simulink model "viertanksystempidstoer"  (Simulink 3.00)
settings: Solver=ode45  StartTime=0.0  StopTime=1800  FixedStep=0.01  RelTol=1e-6  AbsTol=1e-6
undefined symbols (not defined in the file or in its folder): A, A12, A23, A34, A4, g, TN, TV
libraries: simulink3 x1
settings Model: SaveTime=off  SaveOutput=off

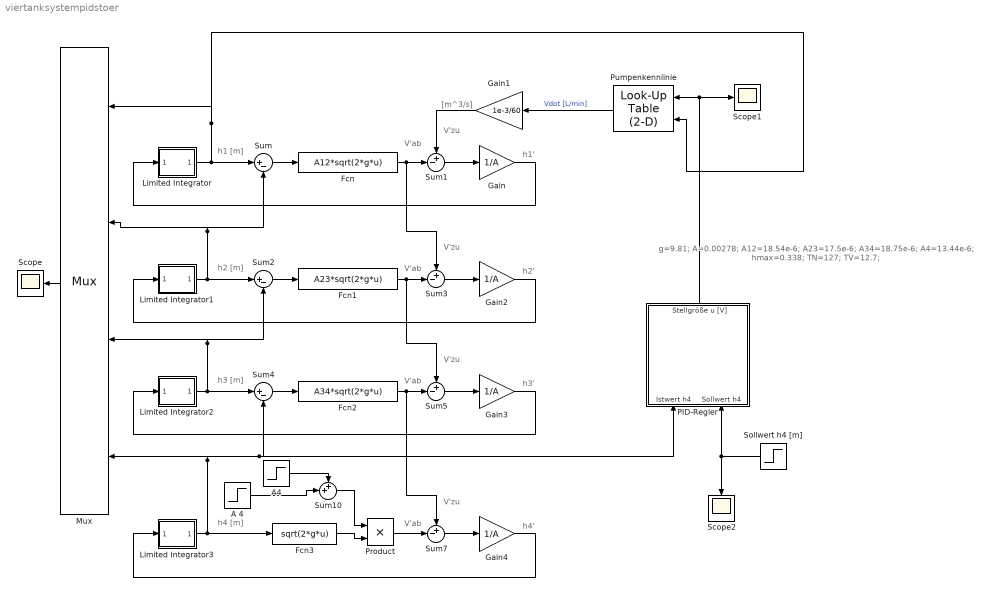
== system viertanksystempidstoer ==
  note: h1 [m]
  note: h1'
  note: [m^3/s]
  note: g=9.81;
      | A=0.00278;
      | A12=18.54e-6;
      | A23=17.5e-6;
      | A34=18.75e-6;
      | A4=13.44e-6;
      | hmax=0.338;
      | TN=127;
      | TV=12.7;
  note: h2 [m]
  note: h2'
  note: V'zu
  note: V'ab
  note: V'zu
  note: V'ab
  note: h3 [m]
  note: h3'
  note: V'zu
  note: V'ab
  note: h4 [m]
  note: h4'
  note: V'zu
  note: V'ab
  A 4 : Step  Time=1230  Before=0  After=A4*0.1749  SampleTime=0
  A4 : Step  Time=600  Before=A4  After=A4*0.8251  SampleTime=0
  Fcn : Fcn  Expr=A12*sqrt(2*g*u)
  Fcn1 : Fcn  Expr=A23*sqrt(2*g*u)
  Fcn2 : Fcn  Expr=A34*sqrt(2*g*u)
  Fcn3 : Fcn  Expr=sqrt(2*g*u)
  Gain{,2..4} (4 alike) : Gain  Gain=1/A  SaturateOnIntegerOverflow=on
  Gain1 : Gain  Orientation=left  Gain=1e-3/60  SaturateOnIntegerOverflow=on
  Limited Integrator : Subsystem  mask(Limited Integrator.){@1=0, @2=hmax, @3=0}
      mask prompts: @1 "Lower bound:"; @2 "Upper bound:"; @3 "Initial condition:"
      mask help: Limited Integrator
      mask init:
      | lower_limit=@1;upper_limit=@2;X0=@3;
      mask Help: Implements a limited integrator with \nan expression of the form:\n\nif(x<=lb and u<0) or (x>=ub and u>0)\n   xdot=0\nelse\n   xdot=u
      mask Display: plot(-1,-0.2,3.5,1.2,[0.05,1,2,2.9],[0,0,1,1]);disp(' 1/s    ')
  Limited Integrator1 : Subsystem  mask(Limited Integrator.){@1=0, @2=hmax, @3=0}
      mask prompts: @1 "Lower bound:"; @2 "Upper bound:"; @3 "Initial condition:"
      mask help: Limited Integrator
      mask init:
      | lower_limit=@1;upper_limit=@2;X0=@3;
      mask Help: Implements a limited integrator with \nan expression of the form:\n\nif(x<=lb and u<0) or (x>=ub and u>0)\n   xdot=0\nelse\n   xdot=u
      mask Display: plot(-1,-0.2,3.5,1.2,[0.05,1,2,2.9],[0,0,1,1]);disp(' 1/s    ')
  Limited Integrator2 : Subsystem  mask(Limited Integrator.){@1=0, @2=hmax, @3=0}
      mask prompts: @1 "Lower bound:"; @2 "Upper bound:"; @3 "Initial condition:"
      mask help: Limited Integrator
      mask init:
      | lower_limit=@1;upper_limit=@2;X0=@3;
      mask Help: Implements a limited integrator with \nan expression of the form:\n\nif(x<=lb and u<0) or (x>=ub and u>0)\n   xdot=0\nelse\n   xdot=u
      mask Display: plot(-1,-0.2,3.5,1.2,[0.05,1,2,2.9],[0,0,1,1]);disp(' 1/s    ')
  Limited Integrator3 : Subsystem  mask(Limited Integrator.){@1=0, @2=hmax, @3=0}
      mask prompts: @1 "Lower bound:"; @2 "Upper bound:"; @3 "Initial condition:"
      mask help: Limited Integrator
      mask init:
      | lower_limit=@1;upper_limit=@2;X0=@3;
      mask Help: Implements a limited integrator with \nan expression of the form:\n\nif(x<=lb and u<0) or (x>=ub and u>0)\n   xdot=0\nelse\n   xdot=u
      mask Display: plot(-1,-0.2,3.5,1.2,[0.05,1,2,2.9],[0,0,1,1]);disp(' 1/s    ')
  Mux : Mux  Orientation=left  Inputs=4
      settings: DisplayOption=none
  PID-Regler : Subsystem  Orientation=up
  Product : Product  Inputs=2  SaturateOnIntegerOverflow=on
  Pumpenkennlinie : simulink3/Functions & Tables/Look-Up Table (2-D)  Orientation=left  x=[ 0 2 3.5 4 6 8 10 12]  y=[ 0 1 2 3 4 5 6 7 8 9 10]*0.338/10  t=[ 0 0 0 0 0 0 0 0 0 0 0 ; 0 0 0 0 0 0 0 0 0 0 0 ; 0.3373 0.2611 0.1115 0.0311 0 0 0 0 0 0 0 ; 0.6051 0.5588 0.5222 0.4851 0.4488 0.3499 0.2844 0.2148 0.1899 0.1431 0.0861; 1.3367 1.3073 1.2845 1.2640 1.2531 1.2297 1.2081 1.1914 1.1831 1.1704 1.1614 ; 1.8718 1.8689 1.8632 1.8579 1.8491 1.8375 1.8271 1.8120 1.8045 1.7843 1.7733 ; 2.4327 2.4253 2.4193 2.4161 2.4095 2.4071 2.4035 2.3993 2.3941 2.3847 2.3799 ; 2.9356 2.9306 2.9291 2.9187 2.9165 2.9125 2.8945 2.8922 2.8855 2.8775 2.8744 ]
  Scope : Scope
      settings: TimeRange=auto  YMin=0.08  YMax=0.18  SaveName=h  DataFormat=Matrix
  Scope1 : Scope
      settings: TimeRange=auto  YMin=7e-034  YMax=2.1e-033  SaveName=up  DataFormat=Matrix
  Scope2 : Scope
      settings: Orientation=down  TimeRange=auto  YMin=-1  YMax=1.1  SaveName=w  DataFormat=Matrix
  Sollwert h4 [m] : Step  Orientation=left  Time=5  Before=0  After=2.5*0.0338  SampleTime=0
  Sum : Sum  Inputs=|+-  SaturateOnIntegerOverflow=on
  Sum{1,3,5,7} (4 alike) : Sum  Inputs=+-|  SaturateOnIntegerOverflow=on
  Sum10 : Sum  Inputs=++|  SaturateOnIntegerOverflow=on
  Sum2 : Sum  Inputs=|+-  SaturateOnIntegerOverflow=on
  Sum4 : Sum  Inputs=|+-  SaturateOnIntegerOverflow=on
  wires:
  Sum/1 -> Fcn/1
  Limited Integrator/1(Outport) -> Sum/1, Mux/1, Pumpenkennlinie/2
  Sum1/1 -> Gain/1
  Gain/1 -> Limited Integrator/1(Inport)
  Gain1/1 -> Sum1/1
  Sum2/1 -> Fcn1/1
  Sum3/1 -> Gain2/1
  Gain2/1 -> Limited Integrator1/1(Inport)
  Limited Integrator1/1(Outport) -> Sum2/1, Sum/2, Mux/2
  Fcn/1 -> Sum1/2, Sum3/1
  Sum4/1 -> Fcn2/1
  Sum5/1 -> Gain3/1
  Gain3/1 -> Limited Integrator2/1(Inport)
  Limited Integrator2/1(Outport) -> Sum4/1, Sum2/2, Mux/3
  Fcn2/1 -> Sum5/2, Sum7/1
  Fcn1/1 -> Sum3/2, Sum5/1
  Pumpenkennlinie/1 -> Gain1/1  "Vdot [L/min]"
  Mux/1 -> Scope/1
  Sum7/1 -> Gain4/1
  Gain4/1 -> Limited Integrator3/1(Inport)
  Limited Integrator3/1(Outport) -> Fcn3/1, Mux/4, Sum4/2, PID-Regler/1(Istwert h4)
  Fcn3/1 -> Product/2
  Product/1 -> Sum7/2
  A4/1 -> Sum10/1
  A 4/1 -> Sum10/2
  Sum10/1 -> Product/1
  PID-Regler/1(Stellgröße u [V]) -> Pumpenkennlinie/1, Scope1/1
  Sollwert h4 [m]/1 -> PID-Regler/2(Sollwert h4), Scope2/1

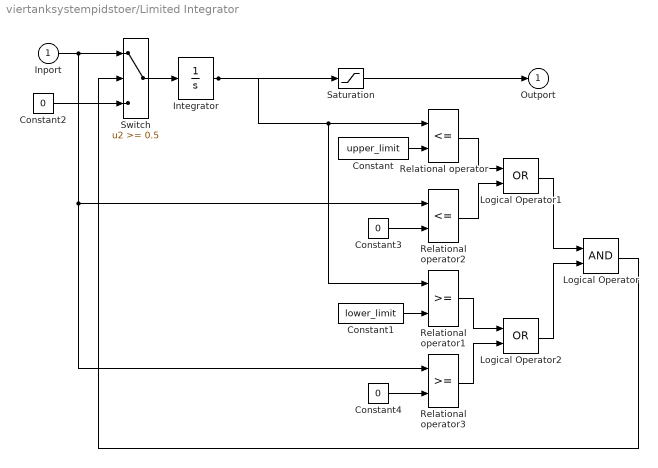
== system viertanksystempidstoer/Limited Integrator ==
  Inport : Inport  Port=1  PortWidth=-1  SampleTime=-1  DataType=auto
      settings: SignalType=auto
  Constant : Constant  Value=upper_limit
  Constant1 : Constant  Value=lower_limit
  Constant2 : Constant  Value=0
  Constant3 : Constant  Value=0
  Constant4 : Constant  Value=0
  Integrator : Integrator  ExternalReset=none  InitialConditionSource=internal  InitialCondition=X0  LimitOutput=off  UpperSaturationLimit=inf  LowerSaturationLimit=-inf  ShowSaturationPort=off  ShowStatePort=off  AbsoluteTolerance=auto
  Logical Operator : Logic  Operator=AND  Inputs=2
  Logical Operator1 : Logic  Operator=OR  Inputs=2
  Logical Operator2 : Logic  Operator=OR  Inputs=2
  Relational operator : RelationalOperator  Operator=<=
  Relational operator1 : RelationalOperator  Operator=>=
  Relational operator2 : RelationalOperator  Operator=<=
  Relational operator3 : RelationalOperator  Operator=>=
  Saturation : Saturate  UpperLimit=upper_limit  LowerLimit=lower_limit
  Switch : Switch  Threshold=0.5
  Outport : Outport  Port=1
  wires:
  Saturation/1 -> Outport/1
  Inport/1 -> Switch/1, Relational operator2/1, Relational operator3/1
  Switch/1 -> Integrator/1
  Constant/1 -> Relational operator/2
  Constant1/1 -> Relational operator1/2
  Logical Operator/1 -> Switch/2
  Constant2/1 -> Switch/3
  Relational operator/1 -> Logical Operator1/1
  Relational operator2/1 -> Logical Operator1/2
  Logical Operator1/1 -> Logical Operator/1
  Relational operator1/1 -> Logical Operator2/1
  Relational operator3/1 -> Logical Operator2/2
  Logical Operator2/1 -> Logical Operator/2
  Constant3/1 -> Relational operator2/2
  Constant4/1 -> Relational operator3/2
  Integrator/1 -> Saturation/1, Relational operator1/1, Relational operator/1

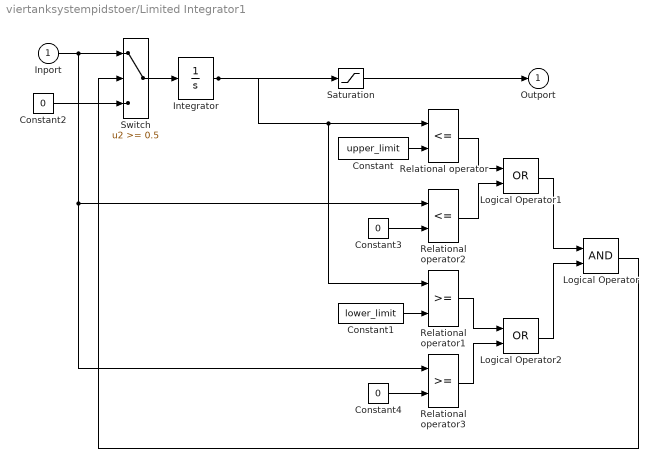
== system viertanksystempidstoer/Limited Integrator1 ==
  Inport : Inport  Port=1  PortWidth=-1  SampleTime=-1  DataType=auto
      settings: SignalType=auto
  Constant : Constant  Value=upper_limit
  Constant1 : Constant  Value=lower_limit
  Constant2 : Constant  Value=0
  Constant3 : Constant  Value=0
  Constant4 : Constant  Value=0
  Integrator : Integrator  ExternalReset=none  InitialConditionSource=internal  InitialCondition=X0  LimitOutput=off  UpperSaturationLimit=inf  LowerSaturationLimit=-inf  ShowSaturationPort=off  ShowStatePort=off  AbsoluteTolerance=auto
  Logical Operator : Logic  Operator=AND  Inputs=2
  Logical Operator1 : Logic  Operator=OR  Inputs=2
  Logical Operator2 : Logic  Operator=OR  Inputs=2
  Relational operator : RelationalOperator  Operator=<=
  Relational operator1 : RelationalOperator  Operator=>=
  Relational operator2 : RelationalOperator  Operator=<=
  Relational operator3 : RelationalOperator  Operator=>=
  Saturation : Saturate  UpperLimit=upper_limit  LowerLimit=lower_limit
  Switch : Switch  Threshold=0.5
  Outport : Outport  Port=1
  wires:
  Integrator/1 -> Relational operator/1, Relational operator1/1, Saturation/1
  Constant4/1 -> Relational operator3/2
  Constant3/1 -> Relational operator2/2
  Logical Operator2/1 -> Logical Operator/2
  Relational operator3/1 -> Logical Operator2/2
  Relational operator1/1 -> Logical Operator2/1
  Logical Operator1/1 -> Logical Operator/1
  Relational operator2/1 -> Logical Operator1/2
  Relational operator/1 -> Logical Operator1/1
  Constant2/1 -> Switch/3
  Logical Operator/1 -> Switch/2
  Constant1/1 -> Relational operator1/2
  Constant/1 -> Relational operator/2
  Switch/1 -> Integrator/1
  Inport/1 -> Relational operator3/1, Relational operator2/1, Switch/1
  Saturation/1 -> Outport/1

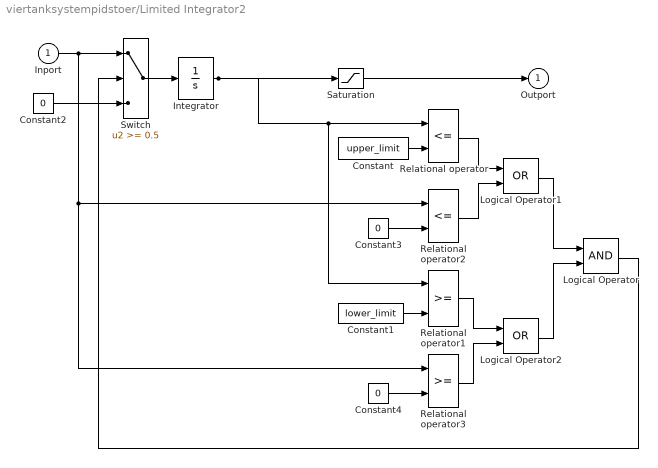
== system viertanksystempidstoer/Limited Integrator2 ==
  Inport : Inport  Port=1  PortWidth=-1  SampleTime=-1  DataType=auto
      settings: SignalType=auto
  Constant : Constant  Value=upper_limit
  Constant1 : Constant  Value=lower_limit
  Constant2 : Constant  Value=0
  Constant3 : Constant  Value=0
  Constant4 : Constant  Value=0
  Integrator : Integrator  ExternalReset=none  InitialConditionSource=internal  InitialCondition=X0  LimitOutput=off  UpperSaturationLimit=inf  LowerSaturationLimit=-inf  ShowSaturationPort=off  ShowStatePort=off  AbsoluteTolerance=auto
  Logical Operator : Logic  Operator=AND  Inputs=2
  Logical Operator1 : Logic  Operator=OR  Inputs=2
  Logical Operator2 : Logic  Operator=OR  Inputs=2
  Relational operator : RelationalOperator  Operator=<=
  Relational operator1 : RelationalOperator  Operator=>=
  Relational operator2 : RelationalOperator  Operator=<=
  Relational operator3 : RelationalOperator  Operator=>=
  Saturation : Saturate  UpperLimit=upper_limit  LowerLimit=lower_limit
  Switch : Switch  Threshold=0.5
  Outport : Outport  Port=1
  wires:
  Saturation/1 -> Outport/1
  Inport/1 -> Switch/1, Relational operator2/1, Relational operator3/1
  Switch/1 -> Integrator/1
  Constant/1 -> Relational operator/2
  Constant1/1 -> Relational operator1/2
  Logical Operator/1 -> Switch/2
  Constant2/1 -> Switch/3
  Relational operator/1 -> Logical Operator1/1
  Relational operator2/1 -> Logical Operator1/2
  Logical Operator1/1 -> Logical Operator/1
  Relational operator1/1 -> Logical Operator2/1
  Relational operator3/1 -> Logical Operator2/2
  Logical Operator2/1 -> Logical Operator/2
  Constant3/1 -> Relational operator2/2
  Constant4/1 -> Relational operator3/2
  Integrator/1 -> Saturation/1, Relational operator1/1, Relational operator/1

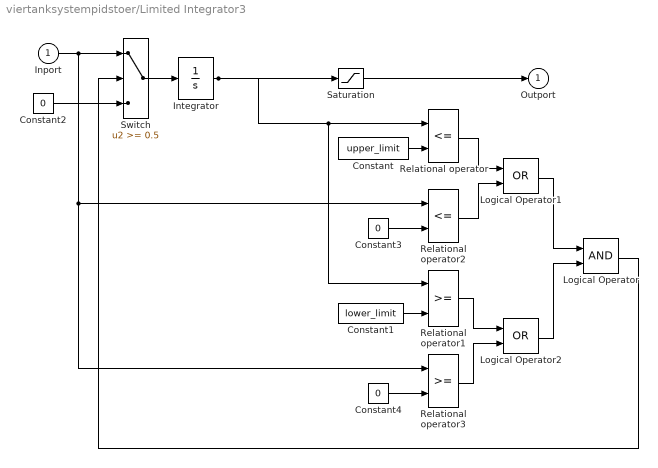
== system viertanksystempidstoer/Limited Integrator3 ==
  Inport : Inport  Port=1  PortWidth=-1  SampleTime=-1  DataType=auto
      settings: SignalType=auto
  Constant : Constant  Value=upper_limit
  Constant1 : Constant  Value=lower_limit
  Constant2 : Constant  Value=0
  Constant3 : Constant  Value=0
  Constant4 : Constant  Value=0
  Integrator : Integrator  ExternalReset=none  InitialConditionSource=internal  InitialCondition=X0  LimitOutput=off  UpperSaturationLimit=inf  LowerSaturationLimit=-inf  ShowSaturationPort=off  ShowStatePort=off  AbsoluteTolerance=auto
  Logical Operator : Logic  Operator=AND  Inputs=2
  Logical Operator1 : Logic  Operator=OR  Inputs=2
  Logical Operator2 : Logic  Operator=OR  Inputs=2
  Relational operator : RelationalOperator  Operator=<=
  Relational operator1 : RelationalOperator  Operator=>=
  Relational operator2 : RelationalOperator  Operator=<=
  Relational operator3 : RelationalOperator  Operator=>=
  Saturation : Saturate  UpperLimit=upper_limit  LowerLimit=lower_limit
  Switch : Switch  Threshold=0.5
  Outport : Outport  Port=1
  wires:
  Integrator/1 -> Relational operator/1, Relational operator1/1, Saturation/1
  Constant4/1 -> Relational operator3/2
  Constant3/1 -> Relational operator2/2
  Logical Operator2/1 -> Logical Operator/2
  Relational operator3/1 -> Logical Operator2/2
  Relational operator1/1 -> Logical Operator2/1
  Logical Operator1/1 -> Logical Operator/1
  Relational operator2/1 -> Logical Operator1/2
  Relational operator/1 -> Logical Operator1/1
  Constant2/1 -> Switch/3
  Logical Operator/1 -> Switch/2
  Constant1/1 -> Relational operator1/2
  Constant/1 -> Relational operator/2
  Switch/1 -> Integrator/1
  Inport/1 -> Relational operator3/1, Relational operator2/1, Switch/1
  Saturation/1 -> Outport/1

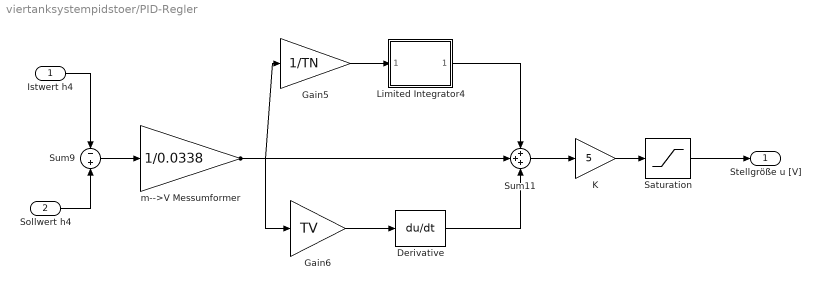
== system viertanksystempidstoer/PID-Regler ==
  Istwert h4 : Inport  Port=1  PortWidth=-1  SampleTime=-1  DataType=auto
      settings: SignalType=auto
  Sollwert h4 : Inport  Port=2  PortWidth=-1  SampleTime=-1  DataType=auto
      settings: SignalType=auto
  Derivative : Derivative
  Gain5 : Gain  Gain=1/TN  SaturateOnIntegerOverflow=on
  Gain6 : Gain  Gain=TV  SaturateOnIntegerOverflow=on
  K : Gain  Gain=5  SaturateOnIntegerOverflow=on
  Limited Integrator4 : Subsystem  mask(Limited Integrator.){@1=0, @2=10, @3=0}
      mask prompts: @1 "Lower bound:"; @2 "Upper bound:"; @3 "Initial condition:"
      mask help: Limited Integrator
      mask init:
      | lower_limit=@1;upper_limit=@2;X0=@3;
      mask Help: Implements a limited integrator with \nan expression of the form:\n\nif(x<=lb and u<0) or (x>=ub and u>0)\n   xdot=0\nelse\n   xdot=u
      mask Display: plot(-1,-0.2,3.5,1.2,[0.05,1,2,2.9],[0,0,1,1]);disp(' 1/s    ')
  Saturation : Saturate  UpperLimit=10  LowerLimit=0
  Sum11 : Sum  Inputs=+++  SaturateOnIntegerOverflow=on
  Sum9 : Sum  Inputs=-|+  SaturateOnIntegerOverflow=on
  m-->V Messumformer : Gain  Gain=1/0.0338  SaturateOnIntegerOverflow=on
  Stellgröße u [V] : Outport  Port=1
  wires:
  Gain5/1 -> Limited Integrator4/1(Inport)
  Gain6/1 -> Derivative/1
  Sum9/1 -> m-->V Messumformer/1
  m-->V Messumformer/1 -> Sum11/2, Gain5/1, Gain6/1
  Istwert h4/1 -> Sum9/1
  Sollwert h4/1 -> Sum9/2
  Limited Integrator4/1(Outport) -> Sum11/1
  Derivative/1 -> Sum11/3
  K/1 -> Saturation/1
  Sum11/1 -> K/1
  Saturation/1 -> Stellgröße u [V]/1

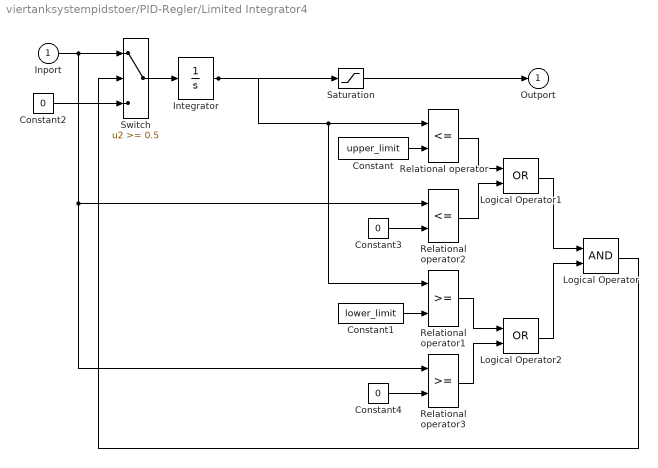
== system viertanksystempidstoer/PID-Regler/Limited Integrator4 ==
  Inport : Inport  Port=1  PortWidth=-1  SampleTime=-1  DataType=auto
      settings: SignalType=auto
  Constant : Constant  Value=upper_limit
  Constant1 : Constant  Value=lower_limit
  Constant2 : Constant  Value=0
  Constant3 : Constant  Value=0
  Constant4 : Constant  Value=0
  Integrator : Integrator  ExternalReset=none  InitialConditionSource=internal  InitialCondition=X0  LimitOutput=off  UpperSaturationLimit=inf  LowerSaturationLimit=-inf  ShowSaturationPort=off  ShowStatePort=off  AbsoluteTolerance=auto
  Logical Operator : Logic  Operator=AND  Inputs=2
  Logical Operator1 : Logic  Operator=OR  Inputs=2
  Logical Operator2 : Logic  Operator=OR  Inputs=2
  Relational operator : RelationalOperator  Operator=<=
  Relational operator1 : RelationalOperator  Operator=>=
  Relational operator2 : RelationalOperator  Operator=<=
  Relational operator3 : RelationalOperator  Operator=>=
  Saturation : Saturate  UpperLimit=upper_limit  LowerLimit=lower_limit
  Switch : Switch  Threshold=0.5
  Outport : Outport  Port=1
  wires:
  Integrator/1 -> Relational operator/1, Relational operator1/1, Saturation/1
  Constant4/1 -> Relational operator3/2
  Constant3/1 -> Relational operator2/2
  Logical Operator2/1 -> Logical Operator/2
  Relational operator3/1 -> Logical Operator2/2
  Relational operator1/1 -> Logical Operator2/1
  Logical Operator1/1 -> Logical Operator/1
  Relational operator2/1 -> Logical Operator1/2
  Relational operator/1 -> Logical Operator1/1
  Constant2/1 -> Switch/3
  Logical Operator/1 -> Switch/2
  Constant1/1 -> Relational operator1/2
  Constant/1 -> Relational operator/2
  Switch/1 -> Integrator/1
  Inport/1 -> Relational operator3/1, Relational operator2/1, Switch/1
  Saturation/1 -> Outport/1
